simulink library "crop_performance_module"  (R2025b)
settings: Solver=VariableStepAuto  StartTime=0.0  StopTime=10.0  RelTol=1e-3
settings Model: Creator=ciepm  LastModifiedBy=charlielenk

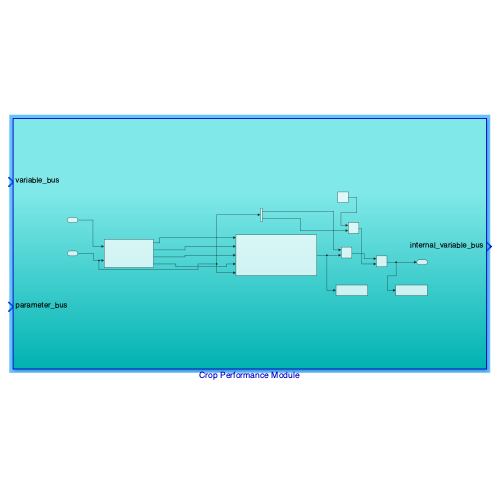
[thumbnail: Simulink's stored preview of the top-level diagram]
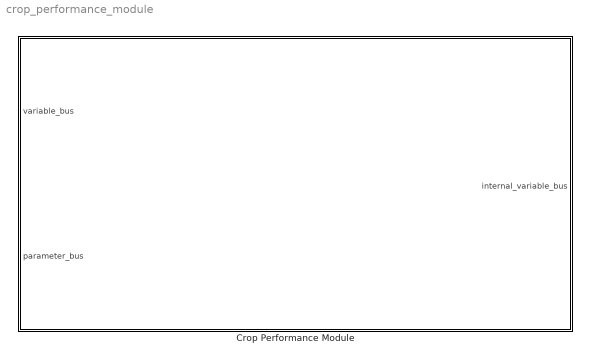
== system crop_performance_module ==
  Crop Performance Module : Subsystem

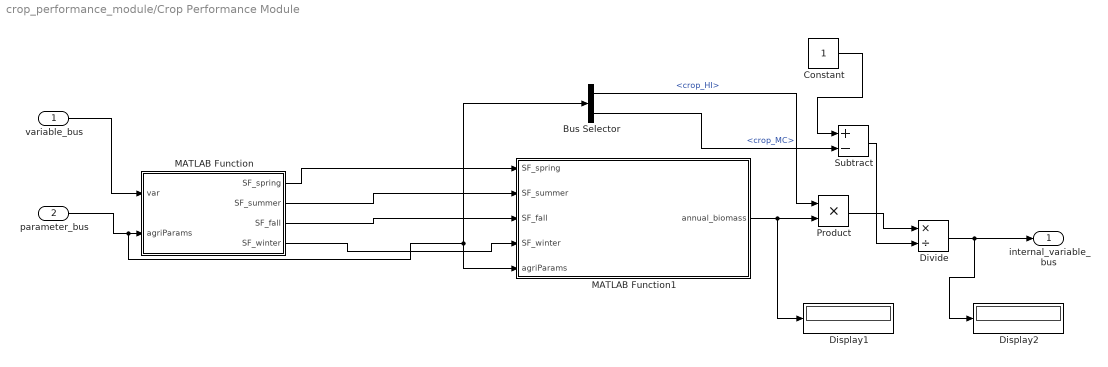
== system crop_performance_module/Crop Performance Module ==
  variable_bus : Inport
  parameter_bus : Inport  Port=2
  Bus Selector : BusSelector  OutputSignals=crop_HI,crop_MC
  Constant : Constant
  Display1 : Display
  Display2 : Display
  Divide : Product  Inputs=*/
  MATLAB Function : MATLAB Function  TreatAsAtomicUnit=on
  MATLAB Function1 : MATLAB Function  TreatAsAtomicUnit=on
  Product : Product
  Subtract : Sum  Inputs=+-
  internal_variable_bus : Outport
  wires:
  Divide/1 -> internal_variable_bus/1, Display2/1
  Subtract/1 -> Divide/2
  Product/1 -> Divide/1
  Bus Selector/2 -> Subtract/2  "<crop_MC>"
  Constant/1 -> Subtract/1
  Bus Selector/1 -> Product/1  "<crop_HI>"
  MATLAB Function1/1(annual_biomass) -> Display1/1, Product/2
  variable_bus/1 -> MATLAB Function/1(var)
  parameter_bus/1 -> MATLAB Function/2(agriParams), MATLAB Function1/5(agriParams), Bus Selector/1
  MATLAB Function/1(SF_spring) -> MATLAB Function1/1(SF_spring)
  MATLAB Function/2(SF_summer) -> MATLAB Function1/2(SF_summer)
  MATLAB Function/3(SF_fall) -> MATLAB Function1/3(SF_fall)
  MATLAB Function/4(SF_winter) -> MATLAB Function1/4(SF_winter)

== matlab function crop_performance_module/Crop Performance Module/MATLAB Function ==
  data: var input; SF_spring output; agriParams input; SF_summer output; SF_fall output; SF_winter output
function [SF_spring, SF_summer, SF_fall, SF_winter] = shading_factor(var, agriParams)
    coder.extrinsic('calculate_shading');

    SF_spring = zeros(24, 1);
    SF_summer = zeros(24, 1);
    SF_fall   = zeros(24, 1);
    SF_winter = zeros(24, 1);

    [SF_spring, SF_summer, SF_fall, SF_winter] = calculate_shading(var, agriParams);
end

== matlab function crop_performance_module/Crop Performance Module/MATLAB Function1 ==
  data: SF_spring input; SF_summer input; SF_fall input; SF_winter input; annual_biomass output; agriParams input
function annual_biomass = crop_growth(SF_spring, SF_summer, SF_fall, SF_winter, agriParams)
    coder.extrinsic('calculate_crop_growth');
    
    annual_biomass = 0;
    % running via function in MATLAB, not simulink (so we can see changes made to funciton in github) 
    annual_biomass = calculate_crop_growth(SF_spring, SF_summer, SF_fall, SF_winter, agriParams);


end
